simulink model "unflipper"  (R2024a)
settings: Solver=ode3  StartTime=0.0  StopTime=Tfinal  FixedStep=step_size  MaxStep=0.001  RelTol=1e-3  EnableMultiTasking=on
values from neighbouring files (symbols this model uses):
  init_cond = [0; 0; 180*pi/180; 0]    [cart_pendulum_model.m]    (also in cart_pendulum_model_angle_only_output.m = [0; 0; 10*pi/180; 0])
  Q = [s1_variance,0,0,0 ... (first row only)    [cart_pendulum_model.m]    (also in cart_pendulum_model_angle_only_output.m; lqr_calcs_2.m = 100*[.5,0,0,0)
  R = [x_variance,0;0,theta_variance]    [cart_pendulum_model.m]    (also in cart_pendulum_model_angle_only_output.m = x_variance; lqr_calcs_2.m = 1)
  s1_variance = .005    (= 0.005)    [cart_pendulum_model.m]    (also in cart_pendulum_model_angle_only_output.m)
  s2_variance = .01    (= 0.01)    [cart_pendulum_model.m]    (also in cart_pendulum_model_angle_only_output.m)
  s3_variance = .05    (= 0.05)    [cart_pendulum_model.m]    (also in cart_pendulum_model_angle_only_output.m)
  s4_variance = .1    (= 0.1)    [cart_pendulum_model.m]    (also in cart_pendulum_model_angle_only_output.m)
  step_size = .01    (= 0.01)    [cart_pendulum_model.m]    (also in cart_pendulum_model_angle_only_output.m)
  theta_variance = 5*pi/180    (= 0.0872664625997)    [cart_pendulum_model.m]    (also in cart_pendulum_model_angle_only_output.m)
  x_variance = .001    (= 0.001)    [cart_pendulum_model.m]
undefined symbols (not defined in the file or in its folder): gaussian, variance
libraries: simulink x6
settings Model: Creator=hurstj  LastModifiedBy=bensor3
settings SolverCC: AlgebraicLoopSolver=TrustRegion
settings DataIOCC: LimitDataPoints=on  SaveFormat=Array  SignalLoggingSaveFormat=ModelDataLogs  ReturnWorkspaceOutputs=off
settings OptimizationCC: BlockReduction=off  DefaultParameterBehavior=Inlined  BufferReuse=off  ExpressionDepthLimit=2147483647  LifeSpan=inf
settings DebuggingCC: UnderspecifiedInitializationDetection=Classic  MergeDetectMultiDrivingBlocksExec=none  SolverPrmCheckMsg=warning  FcnCallInpInsideContextMsg=warning  UnconnectedInputMsg=warning  UnconnectedOutputMsg=warning  UnconnectedLineMsg=warning  StateNameClashWarn=warning  SFUnexpectedBacktrackingDiag=warning  SFNoUnconditionalDefaultTransitionDiag=warning  SFExecutionAtInitializationDiag=none  ArithmeticOperatorsInVariantConditions=warning
settings HardwareCC: ProdBitPerPointer=32  ProdBitPerSizeT=32  ProdBitPerPtrDiffT=32  ProdLargestAtomicFloat=None  ProdIntDivRoundTo=Undefined  ProdEndianess=Unspecified  ProdWordSize=32  ProdHWDeviceType=32-bit Generic
settings ModelReferenceCC: EnableRefExpFcnMdlSchedulingChecks=on  PropagateSignalLabelsOutOfModel=off
settings SFSimCC: SimUseLocalCustomCode=off  CustomCodeUndefinedFunction=UseInterfaceOnly
settings RTWCC: RTWUseLocalCustomCode=off  GPUComputeCapability=3.5  DLArmComputeVersion=19.05
settings CodeAppCC: StateflowObjectComments=on
settings GRTTargetCC: TargetLangStandard=C89/C90 (ANSI)
settings ConfigComp: CovMetricSettings=dw  CovSaveCumulativeToWorkspaceVar=on  CovSaveSingleToWorkspaceVar=on  CovExternalEMLEnable=off

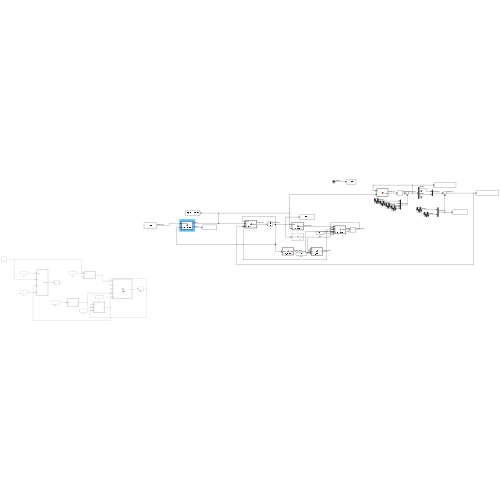
[thumbnail: Simulink's stored preview of the top-level diagram]
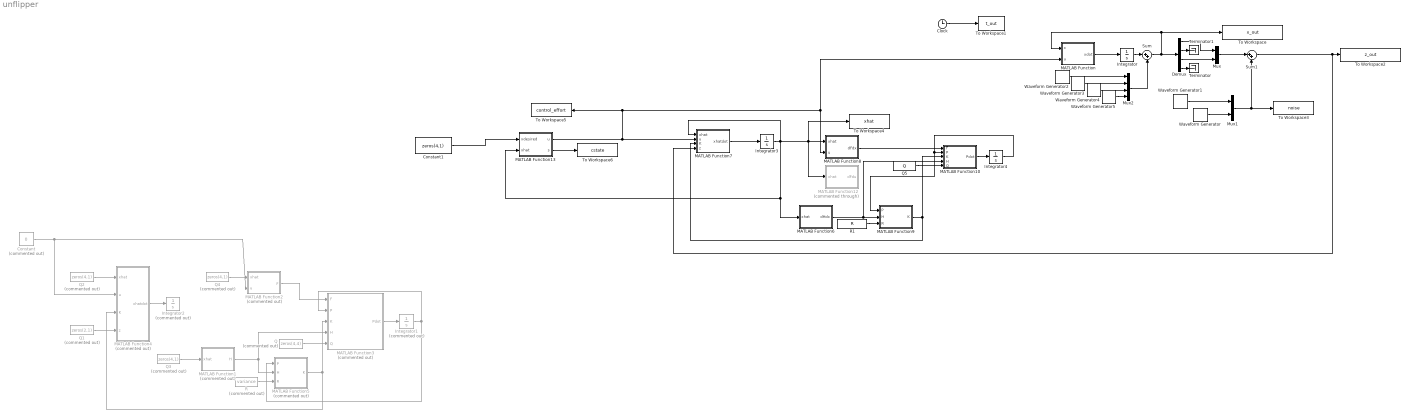
== system unflipper ==
  Clock : Clock
  Constant : Constant  Commented=on  Value=0
  Constant1 : Constant  Value=zeros(4,1)
  Demux : Demux
  Integrator : Integrator  InitialCondition=init_cond
  Integrator1 : Integrator  Commented=on  InitialCondition=zeros(4,4)
  Integrator2 : Integrator  Commented=on  InitialCondition=init_cond
  Integrator3 : Integrator  InitialCondition=init_cond
  Integrator4 : Integrator  InitialCondition=zeros(4,4)
  MATLAB Function : MATLAB Function  TreatAsAtomicUnit=on
  MATLAB Function1 : MATLAB Function  Commented=on  TreatAsAtomicUnit=on
  MATLAB Function10 : MATLAB Function  TreatAsAtomicUnit=on
  MATLAB Function12 : MATLAB Function  Commented=through  TreatAsAtomicUnit=on
  MATLAB Function13 : MATLAB Function  TreatAsAtomicUnit=on
  MATLAB Function2 : MATLAB Function  Commented=on  TreatAsAtomicUnit=on
  MATLAB Function3 : MATLAB Function  Commented=on  TreatAsAtomicUnit=on
  MATLAB Function4 : MATLAB Function  Commented=on  TreatAsAtomicUnit=on
  MATLAB Function5 : MATLAB Function  Commented=on  TreatAsAtomicUnit=on
  MATLAB Function6 : MATLAB Function  TreatAsAtomicUnit=on
  MATLAB Function7 : MATLAB Function  TreatAsAtomicUnit=on
  MATLAB Function8 : MATLAB Function  TreatAsAtomicUnit=on
  MATLAB Function9 : MATLAB Function  TreatAsAtomicUnit=on
  Mux : Mux  Inputs=2
  Mux1 : Mux  Inputs=2
  Mux2 : Mux
  Q : Constant  Commented=on  Value=zeros(4,4)  OutDataTypeStr=Inherit: Inherit via back propagation
  Q1 : Constant  Commented=on  Value=zeros(2,1)  OutDataTypeStr=Inherit: Inherit via back propagation
  Q2 : Constant  Commented=on  Value=zeros(4,1)  OutDataTypeStr=Inherit: Inherit via back propagation
  Q3 : Constant  Commented=on  Value=zeros(4,1)  OutDataTypeStr=Inherit: Inherit via back propagation
  Q4 : Constant  Commented=on  Value=zeros(4,1)  OutDataTypeStr=Inherit: Inherit via back propagation
  Q5 : Constant  Value=Q  OutDataTypeStr=Inherit: Inherit via back propagation
  R : Constant  Commented=on  Value=variance  OutDataTypeStr=Inherit: Inherit via back propagation
  R1 : Constant  Value=R  OutDataTypeStr=Inherit: Inherit via back propagation
  Sum : Sum  Inputs=|++
  Sum1 : Sum  Inputs=|++
  Terminator : Terminator
  Terminator1 : Terminator
  To Workspace : ToWorkspace  VariableName=x_out  SaveFormat=Timeseries  SampleTime=-1
  To Workspace1 : ToWorkspace  VariableName=t_out  SampleTime=-1
  To Workspace2 : ToWorkspace  VariableName=z_out  SaveFormat=Timeseries  SampleTime=-1
  To Workspace3 : ToWorkspace  VariableName=noise  SaveFormat=Timeseries  SampleTime=-1
  To Workspace4 : ToWorkspace  VariableName=xhat  SaveFormat=Timeseries  SampleTime=-1
  To Workspace5 : ToWorkspace  VariableName=control_effort  SaveFormat=Timeseries  SampleTime=-1
  To Workspace6 : ToWorkspace  VariableName=cstate  SaveFormat=Timeseries  SampleTime=-1
  Waveform Generator : simulink/Sources/Waveform Generator  OutMin=[]  OutMax=[]  OutDataTypeStr=double  SelectedSignal=1  Signals=gaussian(0,theta_variance,0)  BlockNames=MultiportSwitch_59a1d59f57604ef  SampleTime=step_size
  Waveform Generator1 : simulink/Sources/Waveform Generator  OutMin=[]  OutMax=[]  OutDataTypeStr=double  SelectedSignal=1  Signals=gaussian(0,x_variance,0)  BlockNames=MultiportSwitch_f67fa682d7ac4fa  SampleTime=step_size
  Waveform Generator2 : simulink/Sources/Waveform Generator  OutMin=[]  OutMax=[]  OutDataTypeStr=double  SelectedSignal=1  Signals=gaussian(0,s1_variance,0)  BlockNames=MultiportSwitch_76d5559e029b4c9  SampleTime=step_size
  Waveform Generator3 : simulink/Sources/Waveform Generator  OutMin=[]  OutMax=[]  OutDataTypeStr=double  SelectedSignal=1  Signals=gaussian(0,s2_variance,0)  BlockNames=MultiportSwitch_7c45e422da1b408  SampleTime=step_size
  Waveform Generator4 : simulink/Sources/Waveform Generator  OutMin=[]  OutMax=[]  OutDataTypeStr=double  SelectedSignal=1  Signals=gaussian(0,s3_variance,0)  BlockNames=MultiportSwitch_9938c4835923451  SampleTime=step_size
  Waveform Generator5 : simulink/Sources/Waveform Generator  OutMin=[]  OutMax=[]  OutDataTypeStr=double  SelectedSignal=1  Signals=gaussian(0,s4_variance,0)  BlockNames=MultiportSwitch_e478b9605acf4b0  SampleTime=step_size
  wires:
  Clock/1 -> To Workspace1/1
  MATLAB Function/1(xdot) -> Integrator/1
  Demux/1 -> Mux/1
  Demux/3 -> Mux/2
  Mux/1 -> Sum1/1
  Sum1/1 -> MATLAB Function7/4(z), To Workspace2/1
  Demux/2 -> Terminator1/1
  Demux/4 -> Terminator/1
  Mux1/1 -> Sum1/2, To Workspace3/1
  Waveform Generator1/1 -> Mux1/1
  Waveform Generator/1 -> Mux1/2
  MATLAB Function3/1(Pdot) -> Integrator1/1
  MATLAB Function4/1(xhatdot) -> Integrator2/1
  R/1 -> MATLAB Function5/3(R)
  MATLAB Function1/1(H) -> MATLAB Function3/4(H), MATLAB Function5/2(H)
  Q/1 -> MATLAB Function3/5(Q)
  MATLAB Function5/1(K) -> MATLAB Function3/3(K), MATLAB Function4/3(K)
  Integrator1/1 -> MATLAB Function5/1(P), MATLAB Function3/2(P)
  Constant/1 -> MATLAB Function2/2(u), MATLAB Function4/2(u)
  Q1/1 -> MATLAB Function4/4(z)
  Q2/1 -> MATLAB Function4/1(xhat)
  Q3/1 -> MATLAB Function1/1(xhat)
  Q4/1 -> MATLAB Function2/1(xhat)
  MATLAB Function2/1(F) -> MATLAB Function3/1(F)
  MATLAB Function10/1(Pdot) -> Integrator4/1
  Integrator4/1 -> MATLAB Function9/1(P), MATLAB Function10/2(P)
  MATLAB Function8/1(dFdx) -> MATLAB Function10/1(F)
  MATLAB Function7/1(xhatdot) -> Integrator3/1
  Integrator3/1 -> MATLAB Function13/2(xhat), MATLAB Function6/1(xhat), MATLAB Function7/1(xhat), MATLAB Function12/1(xhat), To Workspace4/1, MATLAB Function8/1(xhat)
  MATLAB Function6/1(dHdx) -> MATLAB Function10/4(H), MATLAB Function9/2(H)
  R1/1 -> MATLAB Function9/3(R)
  MATLAB Function9/1(K) -> MATLAB Function10/3(K), MATLAB Function7/3(K)
  Q5/1 -> MATLAB Function10/5(Q)
  Integrator/1 -> Sum/1
  Sum/1 -> To Workspace/1, MATLAB Function/1(x), Demux/1
  Mux2/1 -> Sum/2
  Waveform Generator2/1 -> Mux2/1
  Waveform Generator3/1 -> Mux2/2
  Waveform Generator4/1 -> Mux2/3
  Waveform Generator5/1 -> Mux2/4
  MATLAB Function13/1(u) -> To Workspace5/1, MATLAB Function/2(u), MATLAB Function8/2(u), MATLAB Function7/2(u)
  Constant1/1 -> MATLAB Function13/1(xdesired)
  MATLAB Function13/2(s) -> To Workspace6/1

== matlab function unflipper/MATLAB Function12 ==
  data: xhat input; dFdu output
function dFdu = U_func(xhat)

mb=2.3;
mp=1.4;
l=.88;
g=9.8;
Bp=.0178;
Bb=.734;

x1 = xhat(1);
x2 = xhat(2);
x3 = xhat(3);
x4 = xhat(4);

dFdu = [
                                       0;
            1/(- mp*cos(x3)^2 + mb + mp);
                                       0;
cos(x3)/(- l*mp*cos(x3)^2 + l*mb + l*mp)    
];

end

== matlab function unflipper/MATLAB Function13 ==
  data: u output size=1; xdesired input size=4 1; xhat input size=4 1; s output
function [u, s] = controller(xdesired, xhat)
k = zeros(1,4);
if abs(xhat(3))<60*pi/180
    % k_vert
    k = [-7.07106781186547,	-14.8149882763582,	138.635460958818,	38.3060649990405];
else
    % k_down
    k = [70.7106781186554,	49.9686647717991,	-138.382437004899,	14.6020157391927];
end
u = k*(xdesired-xhat);
s = abs(xhat(3))<60*pi/180;
end

== matlab function unflipper/MATLAB Function1 ==
  data: xhat input size=4; H output size=4
function H = H_func(xhat)
H = [1 0 0 0; 0 0 1 0];

end

== matlab function unflipper/MATLAB Function ==
  data: x input size=4; u input; xdot output size=4
function xdot = f(x,u)
xdot=zeros(4,1);
mb=2.3;
mp=1.4;
l=.88;
g=9.8;
Bp=.0178;
Bb=.734;
M=[mp+mb,           -mp*l*cos(x(3));
   -mp*l*cos(x(3)), mp*l^2];
b=[u - mp*l*sin(x(3))*x(4)^2-Bb*x(2);
    mp*g*l*sin(x(3))-Bp*x(4)];
temp=M^-1*b;

xdot(1)=x(2);
xdot(2)=temp(1);
xdot(3)=x(4);
xdot(4)=temp(2);
end

== matlab function unflipper/MATLAB Function2 ==
  data: xhat input size=4; u input; F output size=4
function F = F_func(xhat,u)

mb=2.3;
mp=1.4;
l=.88;
g=9.8;
Bp=.0178;
Bb=.734;

x1 = xhat(1);
x2 = xhat(2);
x3 = xhat(3);
x4 = xhat(4);

dFdx = zeros(4,4);

dFdx(:,1)=[
0;
0;
0;
0];
dFdx(:,2)=[
                                             1;
                -Bb/(- mp*cos(x3)^2 + mb + mp);
                                             0;
-(Bb*cos(x3))/(- l*mp*cos(x3)^2 + l*mb + l*mp)];

dFdx(:,3)=[

                                                                                                                                                                                                                                                                                                                                                                                                                               0;
                                                                       (sin(x3)*(Bp*x4 - g*l*mp*sin(x3)))/(- l*mp*cos(x3)^2 + l*mb + l*mp) + (2*mp*cos(x3)*sin(x3)*(l*mp*sin(x3)*x4^2 - u + Bb*x2))/(- mp*cos(x3)^2 + mb + mp)^2 + (g*l*mp*cos(x3)^2)/(- l*mp*cos(x3)^2 + l*mb + l*mp) - (l*mp*x4^2*cos(x3))/(- mp*cos(x3)^2 + mb + mp) + (2*l*mp*cos(x3)^2*sin(x3)*(Bp*x4 - g*l*mp*sin(x3)))/(- l*mp*cos(x3)^2 + l*mb + l*mp)^2;
                                                                                                                                                                                                                                                                                                                                                                                                                               0;
(sin(x3)*(l*mp*sin(x3)*x4^2 - u + Bb*x2))/(- l*mp*cos(x3)^2 + l*mb + l*mp) - (l*mp*x4^2*cos(x3)^2)/(- l*mp*cos(x3)^2 + l*mb + l*mp) + (2*l*mp*cos(x3)^2*sin(x3)*(l*mp*sin(x3)*x4^2 - u + Bb*x2))/(- l*mp*cos(x3)^2 + l*mb + l*mp)^2 + (g*l*mp*cos(x3)*(mb + mp))/(- l^2*mp^2*cos(x3)^2 + l^2*mp^2 + mb*l^2*mp) + (2*l^2*mp^2*cos(x3)*sin(x3)*(Bp*x4 - g*l*mp*sin(x3))*(mb + mp))/(- l^2*mp^2*cos(x3)^2 + l^2*mp^2 + mb*l^2*mp)^2;
 ];

dFdx(:,4)=[

                                                                                                                            0;
                             - (Bp*cos(x3))/(- l*mp*cos(x3)^2 + l*mb + l*mp) - (2*l*mp*x4*sin(x3))/(- mp*cos(x3)^2 + mb + mp);
                                                                                                                            1;
- (Bp*(mb + mp))/(- l^2*mp^2*cos(x3)^2 + l^2*mp^2 + mb*l^2*mp) - (2*l*mp*x4*cos(x3)*sin(x3))/(- l*mp*cos(x3)^2 + l*mb + l*mp)
 ];
F = dFdx;
end

== matlab function unflipper/MATLAB Function3 ==
  data: F input size=4; P input; K input; H input; Pdot output size=4; Q input
function Pdot = P_func(F,P,K,H,Q)
Pdot = F*P + P*F' - K*H*P+Q;

end

== matlab function unflipper/MATLAB Function4 ==
  data: xhat input size=4; u input; xhatdot output size=4; K input; z input
function xhatdot = xhat_func(xhat,u,K,z)

xdot=zeros(4,1);
mb=2.3;
mp=1.4;
l=.88;
g=9.8;
Bp=.0178;
Bb=.734;
M=[mp+mb,           -mp*l*cos(xhat(3));
   -mp*l*cos(xhat(3)), mp*l^2];
b=[u - mp*l*sin(xhat(3))*xhat(4)^2-Bb*xhat(2);
    mp*g*l*sin(xhat(3))-Bp*xhat(4)];
temp=M^-1*b;

xdot(1)=xhat(2);
xdot(2)=temp(1);
xdot(3)=xhat(4);
xdot(4)=temp(2);

f = xdot;

h = [xhat(1);xhat(3)];
xhatdot = f+K*(z-h);
end

== matlab function unflipper/MATLAB Function5 ==
  data: P input size=4; K output size=4; H input; R input
function K = K_func(P,H,R)

K = P*H'*R^-1;
end

== matlab function unflipper/MATLAB Function6 ==
  data: xhat input; dHdx output
function dHdx = H_func(xhat)

dHdx = [1 0 0 0; 0 0 1 0];

end

== matlab function unflipper/MATLAB Function7 ==
  data: xhat input; u input; xhatdot output; K input; z input
function xhatdot = xhat_func(xhat,u,K,z)

xdot=zeros(4,1);
mb=2.3;
mp=1.4;
l=.88;
g=9.8;
Bp=.0178;
Bb=.734;
M=[mp+mb,           -mp*l*cos(xhat(3));
   -mp*l*cos(xhat(3)), mp*l^2];
b=[u - mp*l*sin(xhat(3))*xhat(4)^2-Bb*xhat(2);
    mp*g*l*sin(xhat(3))-Bp*xhat(4)];
temp=M^-1*b;

xdot(1)=xhat(2);
xdot(2)=temp(1);
xdot(3)=xhat(4);
xdot(4)=temp(2);

f = xdot;

h = [xhat(1);xhat(3)];
xhatdot = f+K*(z-h);
end

== matlab function unflipper/MATLAB Function8 ==
  data: xhat input; u input; dFdx output
function dFdx = F_func(xhat,u)

mb=2.3;
mp=1.4;
l=.88;
g=9.8;
Bp=.0178;
Bb=.734;

x1 = xhat(1);
x2 = xhat(2);
x3 = xhat(3);
x4 = xhat(4);

dFdx = zeros(4,4);

dFdx(:,1)=[
0;
0;
0;
0];
dFdx(:,2)=[
                                             1;
                -Bb/(- mp*cos(x3)^2 + mb + mp);
                                             0;
-(Bb*cos(x3))/(- l*mp*cos(x3)^2 + l*mb + l*mp)];

dFdx(:,3)=[

                                                                                                                                                                                                                                                                                                                                                                                                                               0;
                                                                       (sin(x3)*(Bp*x4 - g*l*mp*sin(x3)))/(- l*mp*cos(x3)^2 + l*mb + l*mp) + (2*mp*cos(x3)*sin(x3)*(l*mp*sin(x3)*x4^2 - u + Bb*x2))/(- mp*cos(x3)^2 + mb + mp)^2 + (g*l*mp*cos(x3)^2)/(- l*mp*cos(x3)^2 + l*mb + l*mp) - (l*mp*x4^2*cos(x3))/(- mp*cos(x3)^2 + mb + mp) + (2*l*mp*cos(x3)^2*sin(x3)*(Bp*x4 - g*l*mp*sin(x3)))/(- l*mp*cos(x3)^2 + l*mb + l*mp)^2;
                                                                                                                                                                                                                                                                                                                                                                                                                               0;
(sin(x3)*(l*mp*sin(x3)*x4^2 - u + Bb*x2))/(- l*mp*cos(x3)^2 + l*mb + l*mp) - (l*mp*x4^2*cos(x3)^2)/(- l*mp*cos(x3)^2 + l*mb + l*mp) + (2*l*mp*cos(x3)^2*sin(x3)*(l*mp*sin(x3)*x4^2 - u + Bb*x2))/(- l*mp*cos(x3)^2 + l*mb + l*mp)^2 + (g*l*mp*cos(x3)*(mb + mp))/(- l^2*mp^2*cos(x3)^2 + l^2*mp^2 + mb*l^2*mp) + (2*l^2*mp^2*cos(x3)*sin(x3)*(Bp*x4 - g*l*mp*sin(x3))*(mb + mp))/(- l^2*mp^2*cos(x3)^2 + l^2*mp^2 + mb*l^2*mp)^2;
 ];

dFdx(:,4)=[

                                                                                                                            0;
                             - (Bp*cos(x3))/(- l*mp*cos(x3)^2 + l*mb + l*mp) - (2*l*mp*x4*sin(x3))/(- mp*cos(x3)^2 + mb + mp);
                                                                                                                            1;
- (Bp*(mb + mp))/(- l^2*mp^2*cos(x3)^2 + l^2*mp^2 + mb*l^2*mp) - (2*l*mp*x4*cos(x3)*sin(x3))/(- l*mp*cos(x3)^2 + l*mb + l*mp)
 ];
end

== matlab function unflipper/MATLAB Function9 ==
  data: P input; K output; H input; R input
function K = K_func(P,H,R)

K = P*H'*R^-1;
end

== matlab function unflipper/MATLAB Function10 ==
  data: F input; Pdot output; P input; K input; H input; Q input
function Pdot = P_func(F,P,K,H,Q)
Pdot = F*P + P*F' - K*H*P+Q;

end
